simulink library "MarIn_blade"  (R2017a)
settings: Solver=VariableStepAuto  StartTime=0.0  StopTime=10.0  RelTol=1e-3
undefined symbols (not defined in the file or in its folder): bladePar, data_wind_mann, eta_init_n, g, k_t1, k_t2, k_w1, k_w2, lw2, m_h, meanWindSpeed, nu_init_b, p_h_dot_init, p_h_init, posCraneTip, posSling_b, posTuggerline_b, posTuggerlineBase_n, sigbuilder_block
undefined symbols (not defined in the file): d_w1, lt1_init
libraries: MarIn_blade x37
(part 1 of 2)
settings Model: Creator=zhengrur  LastModifiedBy=zhengrur

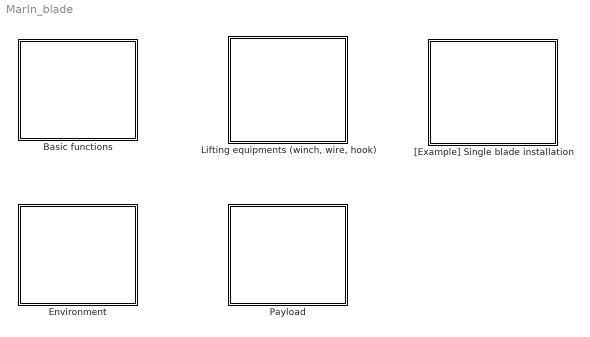
== system MarIn_blade ==
  Basic functions : Subsystem
  Environment : Subsystem
  "Lifting equipments (winch, wire, hook)" : Subsystem
  Payload : Subsystem
  "[Example] Single blade installation" : Subsystem  mask([Example] Single blade installation){}
      mask help:
      | This is an example to use the MarIn toolbox to model single blade installation.
      |
      | Author: Zhengru Ren
      | Date:  19/09/2017

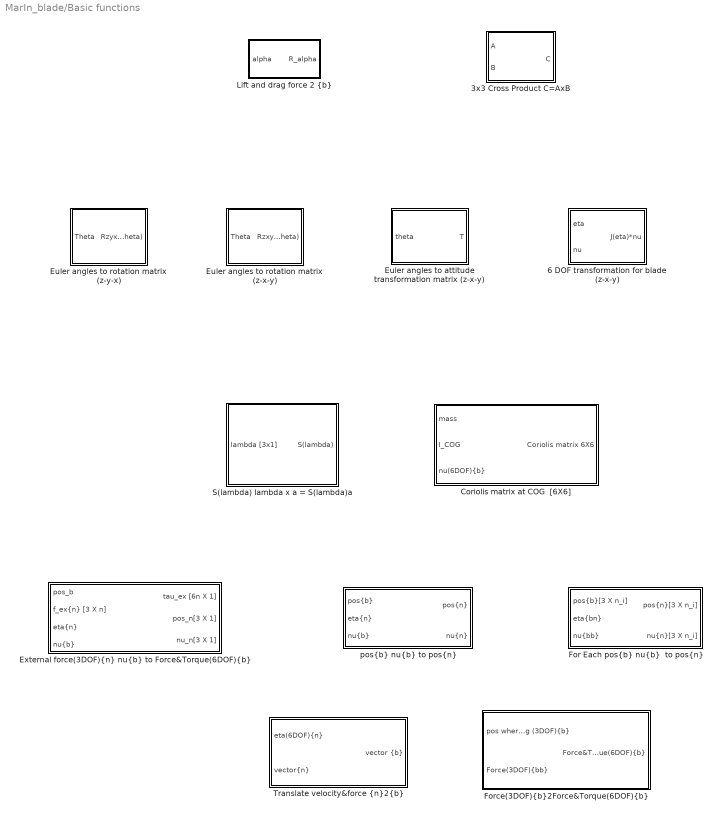
== system MarIn_blade/Basic functions ==
  3x3 Cross Product C=AxB : Subsystem  mask(3x3 Cross Product C=AxB){}
      mask help:
      | [3X1] vector cross product.
      |
      | Author: Zhengru Ren
      | Date: April 22, 2017
  6 DOF transformation for blade (z-x-y) : Subsystem  mask(6 DOF transformation for blade (z-x-y)){}
      mask help:
      | This is an example to use trasform body-fixed velocity to the global frame, with a z-x-y sequence.
      |
      | Author: Zhengru Ren
      | Date:  19/09/2017
  Coriolis matrix at COG  [6X6] : Subsystem  mask(Mass matrix at COG[6X6]){}
      mask help:
      | This block is used to generate the 6X6 mass matrix at the COG.
      |
      |
      | Author: Zhengru Ren
      | Date: April 20, 2017
  Euler angles to rotation matrix (z-x-y) : Subsystem  mask(Euler2R){}
      mask help: Determine the 3-by-3 rotation matrix from the Euler angles (pitch, roll, yaw) using the zxy convention.
      mask Display:
      | port_label('input',1,'theta')
      | port_label('output',1,'R_zxy')
  Euler angles to rotation matrix (z-y-x) : Subsystem  mask(Euler2R){}
      mask help: Determine the 3-by-3 rotation matrix from the Euler angles (roll, pitch, yaw) using the zyx convention.
      mask Display:
      | port_label('input',1,'Theta')
      | port_label('output',1,'R_zyx')
  Euler angles to attitude transformation matrix (z-x-y) : Subsystem  mask(Euler2T){}
      mask help: Determine the 3-by-3 attitude transformation matrix from the Euler angles (roll, pitch, yaw).
      mask Display:
      | port_label('input',1,'Theta')
      | port_label('output',1,'T_zxy')
  "External force(3DOF){n} nu{b} to Force&Torque(6DOF){b}" : Subsystem  mask(External force(3DOF){n} nu{b} to Force&Torque(6DOF){b}){}
      mask help:
      | Translate position and velocity in {b} to {n}.
      |
      |
      | Author: Zhengru Ren
      | Date: April 22, 2017
  "For Each pos{b} nu{b}  to pos{n}" : Subsystem  mask(For Each pos{b} nu{b}  to pos{n}){posCOG_b=bladePar.posCOG, n_i=bladePar.n_i}
      mask prompts: posCOG_b "Position COG {b}"; n_i "number of segment (n_i)"
      mask help:
      | Translate EACH position and velocity in {b} to {n}.
      |
      |
      | Author: Zhengru Ren
      | Date: April 22, 2017
  "Force(3DOF){b}2Force&Torque(6DOF){b}" : Subsystem  mask(Force(3DOF){bb}2Force&Torque(6DOF){bb}){posCOG_bb=bladePar.posCOG}
      mask prompts: posCOG_bb "Position COG {bb}"
      mask help:
      | This block is used to argument a 3DOF force vector to a 6DOF [force;torque] vector.
      |
      |
      |
      |
      | Author: Zhengru Ren
      | Date: April 20, 2017
  "Lift and drag force 2 {b}" : Subsystem  mask(Lift&drag{b}){}
      mask help:
      | The rotational matrix which transformed from the aerodyanmics coordinate to the body-fixed frame.
      |
      | Author: Zhengru Ren
      | Date: April 22, 2017
      mask Display:
      | port_label('input',1,'alpha')
      | port_label('output',1,'R_alpha')
  S(lambda) lambda x a = S(lambda)a : Subsystem  mask(Smatrix){}
      mask help:
      | Output a 3X3 S martix, such that lambda x a = S(lambda)a
      |
      | Author: Zhengru Ren
      | Date: May 10, 2016
  "Translate velocity&force {n}2{b}" : Subsystem  mask(Translate velocity&force {n}2{bb}){}
      mask help:
      | This block is used to transform a 3DOF velcotiy or force vector from {n} to {bb}.
      |
      |
      |
      |
      | Author: Zhengru Ren
      | Date: April 20, 2017
  "pos{b} nu{b} to pos{n}" : Subsystem  TreatAsAtomicUnit=on  mask(pos{bb} to pos{bn} and pos{n}){posCOG_bb=bladePar.posCOG}
      mask prompts: posCOG_bb "Position COG {bb}"
      mask help:
      | Translate the position in {bb} to {bn} and {n}
      |
      |
      | Author: Zhengru Ren
      | Date: April 22, 2017

== system MarIn_blade/Environment ==
  3D wind generator with Mann turbulence : Subsystem  mask(3D wind generator with Mann turbulence){turbulence_switch=on, posC_tb=[0,0,-90], angC_tb=[0,pi,pi/2], data_wind_mann=data_wind_mann}
      mask prompts: turbulence_switch "Turn on the turbulence"; posC_tb "Position of turbulence box center {n}  [X,Y,Z]"; angC_tb "Oritentations of the turbulence box {n} (rad)[phi,theta,psi]"; data_wind_mann "Mann model structure (run init_wind_mann)"
      mask help:
      | This module is used to simulate a wind with Mann turbulence generated from HAWC2 files.
      |
      | Remark: The tubulence will be significantly large if the initial position is not in the turbulence box. For more details, see revelant papers.
      |
      | Author: Zhengru Ren
      | Date: April 18, 2017
      mask Display:
      | image(imread('fig/turbulence.jpg'))
      | 
      | port_label('input', 1, 'Mean wind speed')
      | port_label('input', 2, 'Meansurement point{n}[N x 3]')
      | % port_label('input', 3, 'tau_wind{bb}')
      | 
      | port_label('output', 1, 'wind vel.(3DOF){n}')
      | % port_label('output', 2, 'nuCOG(6DOF){bb}')
      | % port_label('output', 3, 'pCOG(3DOF){n}')
      | % port_label('output', 4, 'pCOG_dot(3DOF){n}')
      | % port_label('output', 5, 'p_i(3DOF){n}')

== system MarIn_blade/Lifting equipments (winch, wire, hook) ==
  Hook : Subsystem  mask(Hook){m_h=m_h, p_h_init=p_h_init, p_h_dot_init=p_h_dot_init}
      mask prompts: m_h "Hook mass (m_h) [kg]"; p_h_init "Initial position of the hook"; p_h_dot_init "Initial velocity of the hook"
      mask help:
      | Used to simulate a hook.
      |
      | Author: Zhengru Ren
      | Date: May 20, 2016
      mask init:
      | invM_h = diag([1/m_h,1/m_h,1/m_h]);
  Winch : Subsystem  mask{l_0=lt1_init}
      mask prompts: l_0 "Initial rope length (m)"
  wire (changable length) : Subsystem  mask(Wire){k=k_w1, c=d_w1}
      mask prompts: k "stiffness (N/m)"; c "damping (Ns/m)"
      mask help:
      | Used to simulate a wire. Tension exists only when the enlongation is larger than 0.
      |
      |
      | Author: Zhengru Ren
      | Date: May 20, 2016
      mask DialogControl DescTextVar Prompt: %<MaskDescription>This module is applied to simulate an elastic rope. When the elongation < 0, there will be no restoring force.

== system MarIn_blade/Payload ==
  Suspended blade : Subsystem  mask(Blade){m_yoke=20e3, bladePar=bladePar, eta_init_n=eta_init_n, eta_init_b=nu_init_b, n_tugline=2, posTuggerline_b=posTuggerline_b, n_sling=2, posSling_b=posSling_b}
      mask prompts: m_yoke "Mass of yoke (kg)"; bladePar "Blade parameter structure"; eta_init_n "Initial position and attitude {n}"; eta_init_b "Initial velocity {b}"; n_tugline "Number of tugger lines (n_tugline)"; posTuggerline_b "Position of connection points to the Tuggerlines{b} [n_tugline x 3]"; n_sling "Number of slings (n_sling)"; posSling_b "Position of connection points to the slings {b} [3Xn_sling]"
      mask help:
      | This block is used to simulate a suspended blade lifted by a crane and control by tuglines.
      |
      |
      | Author: Zhengru Ren
      | Date: April 20, 2017
      mask init:
      | invM_total = inv(bladePar.M+diag([m_yoke,m_yoke,m_yoke,0,0,0]));
      mask Display:
      | image(imread('fig/blade.png'))
      | 
      | port_label('input', 1, 'f_sling1{n}')
      | port_label('input', 2, 'f_sling2{n}')
      | port_label('input', 3, 'f_tagline1{n}')
      | port_label('input', 4, 'f_tagline2{n}')
      | port_label('input', 5, 'tau_wind{b}')
      | 
      | port_label('output', 1, 'etaCOG(6DOF){n}')
      | port_label('output', 2, 'nuCOG(6DOF){b}')
      | port_label('output', 3, 'BUS')
  Wind loads acting on the blade : Subsystem  mask(Wind loads acting on the blade){}
      mask help:
      | This module is used to calculate the wind load acting on a blade in the body frame.
      |
      | Author: Zhengru Ren
      | Date: April 18, 2017
      mask Display:
      | image(imread('fig/blade_coordinate2.png'))
      | 
      | port_label('input', 1, 'eta_n')
      | port_label('input', 2, 'wind vel.{n}[3 x n_i]')
      | port_label('input', 3, 'nu_i{n}[3 x n_i]')
      | % port_label('input', 3, 'tau_wind{bb}')
      | 
      | port_label('output', 1, 'tau_wind{b}')
      | port_label('output', 2, 'BUS')
      | % port_label('output', 2, 'nuCOG(6DOF){bb}')
      | % port_label('output', 3, 'pCOG(3DOF){n}')
      | % port_label('output', 4, 'pCOG_dot(3DOF){n}')
      | % port_label('output', 5, 'p_i(3DOF){n}')

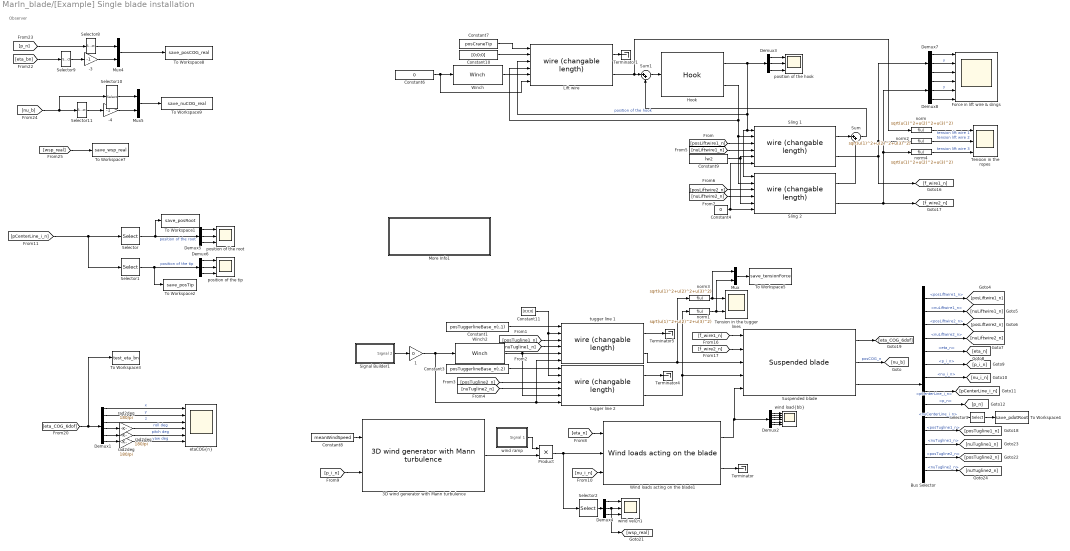
== system MarIn_blade/[Example] Single blade installation ==
  note: Observer
  " rad2deg" : Gain  Gain=180/pi
  -3 : Gain  Gain=-1
  -4 : Gain  Gain=-1
  1 : Gain  Gain=0
  3D wind generator with Mann turbulence : MarIn_blade/Environment/3D wind generator with Mann turbulence  turbulence_switch=on  posC_tb=[0,0,-90]  angC_tb=[0,0,0]  data_wind_mann=data_wind_mann
  Bus Selector : BusSelector  OutputSignals=posLiftwire1_n,nuLiftwire1_n,posLiftwire2_n,nuLiftwire2_n,eta_n,p_i_n,nu_i_n,pCenterLine_i_n,p_n,nuCenterLine_i_n,posTugline1_n,nuTugline1_n,posTugline2_n,nuTugline2_n
  Constant1 : Constant  Value=posTuggerlineBase_n(:,1)
  Constant10 : Constant  Value=[0;0;0]
  Constant11 : Constant  Value=[0;0;0]
  Constant3 : Constant  Value=posTuggerlineBase_n(:,2)
  Constant4 : Constant  Value=0
  Constant6 : Constant  Value=0
  Constant7 : Constant  Value=posCraneTip
  Constant8 : Constant  Value=meanWindSpeed
  Constant9 : Constant  Value=lw2
  Demux1 : Demux  Outputs=6
  Demux2 : Demux  Outputs=6
  Demux{3..8} (6 alike) : Demux  Outputs=3
  Force in lift wire & slings : Scope  NumInputPorts=6
  Hook : MarIn_blade/Lifting equipments (winch, wire, hook)/Hook  m_h=m_h  p_h_init=p_h_init  p_h_dot_init=p_h_dot_init
  Lift wire : MarIn_blade/Lifting equipments (winch, wire, hook)/wire (changable length)  k=k_w1  c=d_w1
  More Info1 : Subsystem
      settings: OpenFcn=run init_example_single_blade_installation.m
      mask Display: disp('Double-click to initialize the model')
  Mux : Mux  Inputs=2
  Mux4 : Mux  Inputs=2
  Mux5 : Mux  Inputs=2
  Product : Product
  Selector : Selector  NumberOfDimensions=2  InputPortWidth=3  IndexOptions=Index vector (dialog),Index vector (dialog)  Indices=[1 2 3],1  OutputSizes=1,1
  Selector1 : Selector  NumberOfDimensions=2  InputPortWidth=3  IndexOptions=Index vector (dialog),Index vector (dialog)  Indices=[1 2 3],bladePar.n_i  OutputSizes=1,1
  Selector10 : Selector  InputPortWidth=6  IndexOptions=Index vector (dialog)  Indices=[3,2]  OutputSizes=1
  Selector11 : Selector  InputPortWidth=6  IndexOptions=Index vector (dialog)  Indices=4  OutputSizes=1
  Selector2 : Selector  NumberOfDimensions=2  InputPortWidth=3  IndexOptions=Index vector (dialog),Index vector (dialog)  Indices=[1 2 3],20  OutputSizes=1,1
  Selector3 : Selector  NumberOfDimensions=2  InputPortWidth=3  IndexOptions=Index vector (dialog),Index vector (dialog)  Indices=[1 2 3],1  OutputSizes=1,1
  Selector8 : Selector  InputPortWidth=3  IndexOptions=Index vector (dialog)  Indices=[1 2]  OutputSizes=1
  Selector9 : Selector  InputPortWidth=6  IndexOptions=Index vector (dialog)  Indices=4  OutputSizes=1
  Signal Builder1 : Subsystem  Tag=STV Subsys  LoadFcn=sigbuilder_block('load');  StartFcn=sigbuilder_block('start');  StopFcn=sigbuilder_block('stop');  ClipboardFcn=sigbuilder_block('clipboard');  mask(Sigbuilder block){tuvar=[0:10]}
      mask help: Simulink:masks:SigbuilderBlock_MD
      mask init:
      | if ~strcmp(get_param(bdroot(gcbh),'SimulationStatus'),'stopped') tuvar = sigbuilder_block('maskInit'); end
      settings: CopyFcn=sigbuilder_block('copy');  DeleteFcn=sigbuilder_block('delete');  ModelCloseFcn=sigbuilder_block('modelClose');  PreSaveFcn=sigbuilder_block('preSave');  PauseFcn=sigbuilder_block('pause');  ContinueFcn=sigbuilder_block('continue');  NameChangeFcn=sigbuilder_block('namechange');  OpenFcn=sigbuilder_block('open',[6 30 1908 951.75 ]);  CloseFcn=sigbuilder_block('close');
      mask Display: plot(0, 0, 100, 100,[2, 2, 32, 32, 2], [68, 8, 8, 68, 68],[32, 2], [38, 38], [32, 19, 2],[53, 60, 44], [32, 17, 17, 2],[16, 16, 31, 31]);txt = getActiveGroup(gcbh);text(2, 100, txt,'verticalAlignment', 'top');
  Sling 1 : MarIn_blade/Lifting equipments (winch, wire, hook)/wire (changable length)  k=k_w2  c=d_w2
  Sling 2 : MarIn_blade/Lifting equipments (winch, wire, hook)/wire (changable length)  k=k_w2  c=d_w2
  Sum : Sum  Inputs=|++
  Sum1 : Sum  Inputs=|++
  Suspended blade : MarIn_blade/Payload/Suspended blade  m_yoke=20e3  bladePar=bladePar  eta_init_n=eta_init_n  eta_init_b=nu_init_b  n_tugline=2  posTuggerline_b=posTuggerline_b  n_sling=2  posSling_b=posSling_b
  Tension in the ropes : Scope  NumInputPorts=3
  Tension in the tugger lines : Scope  NumInputPorts=2
  Terminator{,1,4..5} (4 alike) : Terminator
  To Workspace1 : ToWorkspace  VariableName=save_posRoot  SaveFormat=Structure With Time  SampleTime=-1
  To Workspace2 : ToWorkspace  VariableName=save_posTip  SaveFormat=Structure With Time  SampleTime=-1
  To Workspace3 : ToWorkspace  VariableName=test_eta_bn  SaveFormat=Structure With Time  SampleTime=-1
  To Workspace4 : ToWorkspace  VariableName=save_pdotRoot  SaveFormat=Structure With Time  SampleTime=-1
  To Workspace5 : ToWorkspace  VariableName=save_tensionForce  SaveFormat=Structure With Time  SampleTime=-1
  To Workspace7 : ToWorkspace  VariableName=save_wsp_real  SaveFormat=Structure With Time  SampleTime=-1
  To Workspace8 : ToWorkspace  VariableName=save_posCOG_real  SaveFormat=Structure With Time  SampleTime=-1
  To Workspace9 : ToWorkspace  VariableName=save_nuCOG_real  SaveFormat=Structure With Time  SampleTime=-1
  Winch : MarIn_blade/Lifting equipments (winch, wire, hook)/Winch  l_0=lw1_init
  Winch2 : MarIn_blade/Lifting equipments (winch, wire, hook)/Winch  l_0=lt1_init
  Wind loads acting on the blade1 : MarIn_blade/Payload/Wind loads acting on the blade
      link override "Wind loads acting on node i/Lift and drag force 2 {b}": SourceBlock=MarIn_blade/Basic functions/Lift and drag force 2 {b}
  "etaCOG{n}" : Scope  NumInputPorts=6
  norm{,1..4} (5 alike) : Fcn  Expr=sqrt(u(1)^2+u(2)^2+u(3)^2)
  position of the hook : Scope  NumInputPorts=3
  position of the root : Scope  NumInputPorts=3
  position of the tip : Scope  NumInputPorts=3
  rad2deg : Gain  Gain=180/pi
  "rad2deg " : Gain  Gain=180/pi
  tugger line 1 : MarIn_blade/Lifting equipments (winch, wire, hook)/wire (changable length)  k=k_t1  c=d_t1
  tugger line 2 : MarIn_blade/Lifting equipments (winch, wire, hook)/wire (changable length)  k=k_t2  c=d_t2
  "wind load{bb}" : Scope  NumInputPorts=6
  wind ramp : Subsystem  Tag=STV Subsys  LoadFcn=sigbuilder_block('load');  StartFcn=sigbuilder_block('start');  StopFcn=sigbuilder_block('stop');  ClipboardFcn=sigbuilder_block('clipboard');  mask(Sigbuilder block){tuvar=[0:10]}
      mask help: Simulink:masks:SigbuilderBlock_MD
      mask init:
      | if ~strcmp(get_param(bdroot(gcbh),'SimulationStatus'),'stopped') tuvar = sigbuilder_block('maskInit'); end
      settings: CopyFcn=sigbuilder_block('copy');  DeleteFcn=sigbuilder_block('delete');  ModelCloseFcn=sigbuilder_block('modelClose');  PreSaveFcn=sigbuilder_block('preSave');  PauseFcn=sigbuilder_block('pause');  ContinueFcn=sigbuilder_block('continue');  NameChangeFcn=sigbuilder_block('namechange');  OpenFcn=sigbuilder_block('open',[6 30 1908 951.75 ]);  CloseFcn=sigbuilder_block('close');
      mask Display: plot(0, 0, 100, 100,[2, 2, 32, 32, 2], [68, 8, 8, 68, 68],[32, 2], [38, 38], [32, 19, 2],[53, 60, 44], [32, 17, 17, 2],[16, 16, 31, 31]);txt = getActiveGroup(gcbh);text(2, 100, txt,'verticalAlignment', 'top');
  "wind vel{n}" : Scope  NumInputPorts=3
  wires:
  Constant8/1 -> 3D wind generator with Mann turbulence/1
  Hook/2 -> Lift wire/4, Sling 2/2, Sling 1/2
  Sling 1/1 -> Sum/1
  Winch/1 -> Lift wire/5
  [eta_COG_6dof] -> To Workspace3/1, Demux1/1
  Demux1/5 -> rad2deg/1
  Demux1/4 -> "rad2deg "/1
  Demux2/1 -> "wind load{bb}"/1
  Demux2/2 -> "wind load{bb}"/2
  Demux2/3 -> "wind load{bb}"/3
  Wind loads acting on the blade1/2 -> Terminator/1
  Suspended blade/3 -> Bus Selector/1
  [p_i_n] -> 3D wind generator with Mann turbulence/2
  [posLiftwire1_n] -> Sling 1/3
  [eta_n] -> Wind loads acting on the blade1/1
  Sling 1/2 -> [f_wire1_n], Demux7/1, norm2/1
  [nuLiftwire1_n] -> Sling 1/4
  Suspended blade/2 -> [nu_b]  "posCOG_n"
  Demux2/4 -> "wind load{bb}"/4
  Demux2/5 -> "wind load{bb}"/5
  norm/1 -> Tension in the ropes/1  "tension lift wire 1"
  Demux2/6 -> "wind load{bb}"/6
  [nu_i_n] -> Wind loads acting on the blade1/3
  Sling 2/1 -> Sum/2
  Sling 2/2 -> [f_wire2_n], Demux8/1, norm4/1
  [posLiftwire2_n] -> Sling 2/3
  [nuLiftwire2_n] -> Sling 2/4
  Constant9/1 -> Sling 1/5, Sling 2/5
  Constant7/1 -> Lift wire/1
  Constant10/1 -> Lift wire/2
  Sum/1 -> Sum1/2
  Lift wire/2 -> norm/1, Sum1/1
  Lift wire/1 -> Terminator1/1
  Sum1/1 -> Hook/1
  norm2/1 -> Tension in the ropes/2  "tension lift wire 2"
  norm4/1 -> Tension in the ropes/3  "tension lift wire 3"
  Demux3/1 -> position of the hook/1
  Demux3/3 -> position of the hook/3
  Demux3/2 -> position of the hook/2
  Hook/1 -> Lift wire/3, Sling 2/1, Sling 1/1, Demux3/1  "position of the hook"
  Demux4/1 -> "wind vel{n}"/1
  Demux4/3 -> "wind vel{n}"/3
  Selector2/1 -> Demux4/1
  Demux5/1 -> position of the root/1
  Demux5/3 -> position of the root/3
  Demux5/2 -> position of the root/2
  Selector/1 -> Demux5/1, To Workspace1/1  "position of the root"
  Demux6/1 -> position of the tip/1
  Demux6/3 -> position of the tip/3
  Demux6/2 -> position of the tip/2
  Selector1/1 -> To Workspace2/1, Demux6/1  "position of the tip"
  Demux7/3 -> Force in lift wire & slings/3
  Demux7/2 -> Force in lift wire & slings/2  "y"
  Demux7/1 -> Force in lift wire & slings/1
  Demux8/3 -> Force in lift wire & slings/6
  Demux8/2 -> Force in lift wire & slings/5  "y"
  Demux8/1 -> Force in lift wire & slings/4
  [pCenterLine_i_n] -> Selector1/1, Selector/1
  Constant4/1 -> Sling 2/6, Sling 1/6
  Constant6/1 -> Lift wire/6, Winch/1
  Product/1 -> Wind loads acting on the blade1/2, Selector2/1
  wind ramp/1(Signal 1) -> Product/1
  Demux4/2 -> "wind vel{n}"/2, [wsp_real]
  tugger line 1/2 -> Suspended blade/3, norm3/1
  tugger line 2/2 -> Suspended blade/4, norm1/1
  Demux1/6 -> " rad2deg"/1
  Bus Selector/1 -> [posLiftwire1_n]  "<posLiftwire1_n>"
  Bus Selector/2 -> [nuLiftwire1_n]  "<nuLiftwire1_n>"
  Bus Selector/3 -> [posLiftwire2_n]  "<posLiftwire2_n>"
  Bus Selector/4 -> [nuLiftwire2_n]  "<nuLiftwire2_n>"
  Bus Selector/5 -> [eta_n]  "<eta_n>"
  Bus Selector/6 -> [p_i_n]  "<p_i_n>"
  Bus Selector/7 -> [nu_i_n]  "<nu_i_n>"
  Bus Selector/8 -> [pCenterLine_i_n]  "<pCenterLine_i_n>"
  Bus Selector/9 -> [p_n]  "<p_n>"
  [f_wire1_n] -> Suspended blade/1
  [f_wire2_n] -> Suspended blade/2
  Suspended blade/1 -> [eta_COG_6dof]
  Bus Selector/10 -> Selector3/1  "<nuCenterLine_i_n>"
  Selector3/1 -> To Workspace4/1
  Winch2/1 -> tugger line 2/5, tugger line 1/5
  Constant1/1 -> tugger line 1/1
  Constant3/1 -> tugger line 2/1
  Constant11/1 -> tugger line 2/2, tugger line 1/2
  Signal Builder1/1(Signal 2) -> 1/1
  1/1 -> Winch2/1, tugger line 2/6, tugger line 1/6
  Bus Selector/11 -> [posTugline1_n]  "<posTugline1_n>"
  Bus Selector/13 -> [posTugline2_n]  "<posTugline2_n>"
  Bus Selector/12 -> [nuTugline1_n]  "<nuTugline1_n>"
  Bus Selector/14 -> [nuTugline2_n]  "<nuTugline2_n>"
  [posTugline1_n] -> tugger line 1/3
  [nuTugline1_n] -> tugger line 1/4
  [posTugline2_n] -> tugger line 2/3
  [nuTugline2_n] -> tugger line 2/4
  tugger line 1/1 -> Terminator5/1
  tugger line 2/1 -> Terminator4/1
  norm3/1 -> Mux/1, Tension in the tugger lines/1
  norm1/1 -> Mux/2, Tension in the tugger lines/2
  Mux/1 -> To Workspace5/1
  Selector9/1 -> -3/1
  Selector8/1 -> Mux4/1
  -3/1 -> Mux4/2
  Selector10/1 -> Mux5/1
  Selector11/1 -> -4/1
  -4/1 -> Mux5/2
  Mux5/1 -> To Workspace9/1
  Mux4/1 -> To Workspace8/1
  [eta_bn] -> Selector9/1
  [p_n] -> Selector8/1
  [nu_b] -> Selector11/1, Selector10/1
  [wsp_real] -> To Workspace7/1
  3D wind generator with Mann turbulence/1 -> Product/2
  Demux1/2 -> "etaCOG{n}"/2  "y"
  Demux1/1 -> "etaCOG{n}"/1  "x"
  Demux1/3 -> "etaCOG{n}"/3  "z"
  "rad2deg "/1 -> "etaCOG{n}"/4  "roll deg"
  " rad2deg"/1 -> "etaCOG{n}"/6  "yaw deg"
  rad2deg/1 -> "etaCOG{n}"/5  "pitch deg"
  Wind loads acting on the blade1/1 -> Suspended blade/5, Demux2/1

== system MarIn_blade/Basic functions/3x3 Cross Product C=AxB ==
  A : Inport
  B : Inport  Port=2
  "A " : InportShadow
  "B " : InportShadow  Port=2
  Subsystem2 : Subsystem
  Subsystem3 : Subsystem
  Sum : Sum  Inputs=+|-  SaturateOnIntegerOverflow=on  InputSameDT=on  OutDataTypeStr=Inherit: Same as first input
  C : Outport
  wires:
  "B "/1 -> Subsystem3/2(B)
  "A "/1 -> Subsystem3/1(A)
  Sum/1 -> C/1
  B/1 -> Subsystem2/2(B)
  A/1 -> Subsystem2/1(A)
  Subsystem2/1(Out1) -> Sum/1
  Subsystem3/1(Out1) -> Sum/2

== system MarIn_blade/Basic functions/6 DOF transformation for blade (z-x-y) ==
  note: Theta
  note: v
  note: omega
  eta : Inport
  nu : Inport  Port=2
  Euler angles to rotation matrix (z-x-y) : MarIn_blade/Basic functions/Euler angles to rotation matrix (z-x-y)
      settings: SourceProductName=MarIn(Blade)
  Euler angles to attitude transformation matrix (z-x-y) : MarIn_blade/Basic functions/Euler angles to attitude transformation matrix (z-x-y)
      settings: SourceProductName=MarIn(Blade)
  Mux : Mux  Inputs=2
  Product : Product  Inputs=**  Multiplication=Matrix(*)  SaturateOnIntegerOverflow=on  OutDataTypeStr=Inherit: Same as first input
  Product1 : Product  Inputs=**  Multiplication=Matrix(*)  SaturateOnIntegerOverflow=on  OutDataTypeStr=Inherit: Same as first input
  Selector : Selector  InputPortWidth=6  IndexOptions=Index vector (dialog)  Indices=[4 5 6]  OutputSizes=1
  Selector1 : Selector  InputPortWidth=6  IndexOptions=Index vector (dialog)  Indices=[1 2 3]  OutputSizes=1
  Selector2 : Selector  InputPortWidth=6  IndexOptions=Index vector (dialog)  Indices=[4 5 6]  OutputSizes=1
  J(eta)*nu : Outport
  wires:
  Product/1 -> Mux/1
  Selector/1 -> Euler angles to attitude transformation matrix (z-x-y)/1, Euler angles to rotation matrix (z-x-y)/1
  eta/1 -> Selector/1
  Euler angles to rotation matrix (z-x-y)/1 -> Product/1
  nu/1 -> Selector1/1, Selector2/1
  Selector1/1 -> Product/2
  Selector2/1 -> Product1/2
  Euler angles to attitude transformation matrix (z-x-y)/1 -> Product1/1
  Mux/1 -> J(eta)*nu/1
  Product1/1 -> Mux/2

== system MarIn_blade/Basic functions/Coriolis matrix at COG  [6X6] ==
  mass : Inport
  I_COG : Inport  Port=2
  "nu(6DOF){b}" : Inport  Port=3
  Gain : Gain  Gain=-1
  Overwrite Values [1:3,1:3] : S-Function  FunctionName=sdspoverwrite  Parameters=ColSpan, ColStartMode, ColStartIndex, ColEndMode, ColEndIndex, RowSpan, RowStartMode, RowStartIndex, RowEndMode, RowEndIndex, OverWriteDiag, ConstValue, DiagSpan, DiagStartMode, DiagStartIndex, DiagEndMode, DiagEndIndex, valFrom2ndIP  SFunctionDeploymentMode=off  EnableBusSupport=off  mask(Overwrite Values){OverWriteDiag=Submatrix, valFrom2ndIP=Second input port, ConstValue=0, RowSpan=Range of rows, RowStartMode=Index, RowStartIndex=1, RowEndMode=Index, RowEndIndex=3, ColSpan=Range of columns, ColStartMode=Index, ColStartIndex=1, ColEndMode=Index, ColEndIndex=3, DiagSpan=Range of elements, DiagStartMode=Index, DiagStartIndex=1, DiagEndMode=Index, DiagEndIndex=3}
      mask prompts: OverWriteDiag "Overwrite:"; valFrom2ndIP "Source of overwriting value(s):"; ConstValue "Overwrite with:"; RowSpan "Row span:"; RowStartMode "Starting row:"; RowStartIndex "Starting row index:"; RowEndMode "Ending row:"; RowEndIndex "Ending row index:"; ColSpan "Column span:"; ColStartMode "Starting column:"; ColStartIndex "Starting column index:"; ColEndMode "Ending column:"; ColEndIndex "Ending column index:"; DiagSpan "Diagonal span:"; DiagStartMode "Starting element:"; DiagStartIndex "Starting element index:"; DiagEndMode "Ending element:"; DiagEndIndex "Ending element index:"
      mask help:
      | Overwrites a selected portion of the input matrix--either a submatrix, full diagonal, or a portion of the diagonal.
      | Specify overwriting values as follows:
      |   --Matrix with the same dimensions as the submatrix
      |   --Vector with the same length as the portion of the diagonal
      |   --Scalar constant with which to replace each element in the submatrix or diagonal portion.
      |
      | Treats unoriented (1-D) input vectors as column vectors.
      mask init:
      | [x1,y1,xc,yc,xmc,ymc,xi,yi] = dspblkoverwrite('icon');
      | if valFrom2ndIP == 1
      |   i1=1;
      |   s1='';
      | else
      |   i1=2;
      |   s1='V';
      | end;
      mask Help: eval('blocksethelp');
      mask TypeOptions OverWriteDiag: Submatrix | Diagonal
      mask Callback OverWriteDiag: dspblkoverwrite
      mask TypeOptions valFrom2ndIP: Specify via dialog | Second input port
      mask Callback valFrom2ndIP: dspblkoverwrite
      mask TypeOptions RowSpan: All rows | One row | Range of rows
      mask Callback RowSpan: dspblkoverwrite
      mask TypeOptions RowStartMode: First | Index | Offset from last | Last | Offset from middle | Middle
      mask Callback RowStartMode: dspblkoverwrite
      mask TypeOptions RowEndMode: Index | Offset from last | Last | Offset from middle | Middle
      mask Callback RowEndMode: dspblkoverwrite
      mask TypeOptions ColSpan: All columns | One column | Range of columns
      mask Callback ColSpan: dspblkoverwrite
      mask TypeOptions ColStartMode: First | Index | Offset from last | Last | Offset from middle | Middle
      mask Callback ColStartMode: dspblkoverwrite
      mask TypeOptions ColEndMode: Index | Offset from last | Last | Offset from middle | Middle
      mask Callback ColEndMode: dspblkoverwrite
      mask TypeOptions DiagSpan: All elements | One element | Range of elements
      mask Callback DiagSpan: dspblkoverwrite
      mask TypeOptions DiagStartMode: First | Index | Offset from last | Last | Offset from middle | Middle
      mask Callback DiagStartMode: dspblkoverwrite
      mask TypeOptions DiagEndMode: Index | Offset from last | Last | Offset from middle | Middle
      mask Callback DiagEndMode: dspblkoverwrite
      mask Display:
      | plot(x1,y1,xc,yc,xmc,ymc,xi,yi);
      | port_label('input',1,'A');
      | port_label('output',1,'B');
      | port_label('input',i1,s1);
  Overwrite Values [4:6,4:6] : S-Function  FunctionName=sdspoverwrite  Parameters=ColSpan, ColStartMode, ColStartIndex, ColEndMode, ColEndIndex, RowSpan, RowStartMode, RowStartIndex, RowEndMode, RowEndIndex, OverWriteDiag, ConstValue, DiagSpan, DiagStartMode, DiagStartIndex, DiagEndMode, DiagEndIndex, valFrom2ndIP  SFunctionDeploymentMode=off  EnableBusSupport=off  mask(Overwrite Values){OverWriteDiag=Submatrix, valFrom2ndIP=Second input port, ConstValue=0, RowSpan=Range of rows, RowStartMode=Index, RowStartIndex=4, RowEndMode=Index, RowEndIndex=6, ColSpan=Range of columns, ColStartMode=Index, ColStartIndex=4, ColEndMode=Index, ColEndIndex=6, DiagSpan=Range of elements, DiagStartMode=Index, DiagStartIndex=2, DiagEndMode=Index, DiagEndIndex=4}
      mask prompts: OverWriteDiag "Overwrite:"; valFrom2ndIP "Source of overwriting value(s):"; ConstValue "Overwrite with:"; RowSpan "Row span:"; RowStartMode "Starting row:"; RowStartIndex "Starting row index:"; RowEndMode "Ending row:"; RowEndIndex "Ending row index:"; ColSpan "Column span:"; ColStartMode "Starting column:"; ColStartIndex "Starting column index:"; ColEndMode "Ending column:"; ColEndIndex "Ending column index:"; DiagSpan "Diagonal span:"; DiagStartMode "Starting element:"; DiagStartIndex "Starting element index:"; DiagEndMode "Ending element:"; DiagEndIndex "Ending element index:"
      mask help:
      | Overwrites a selected portion of the input matrix--either a submatrix, full diagonal, or a portion of the diagonal.
      | Specify overwriting values as follows:
      |   --Matrix with the same dimensions as the submatrix
      |   --Vector with the same length as the portion of the diagonal
      |   --Scalar constant with which to replace each element in the submatrix or diagonal portion.
      |
      | Treats unoriented (1-D) input vectors as column vectors.
      mask init:
      | [x1,y1,xc,yc,xmc,ymc,xi,yi] = dspblkoverwrite('icon');
      | if valFrom2ndIP == 1
      |   i1=1;
      |   s1='';
      | else
      |   i1=2;
      |   s1='V';
      | end;
      mask Help: eval('blocksethelp');
      mask TypeOptions OverWriteDiag: Submatrix | Diagonal
      mask Callback OverWriteDiag: dspblkoverwrite
      mask TypeOptions valFrom2ndIP: Specify via dialog | Second input port
      mask Callback valFrom2ndIP: dspblkoverwrite
      mask TypeOptions RowSpan: All rows | One row | Range of rows
      mask Callback RowSpan: dspblkoverwrite
      mask TypeOptions RowStartMode: First | Index | Offset from last | Last | Offset from middle | Middle
      mask Callback RowStartMode: dspblkoverwrite
      mask TypeOptions RowEndMode: Index | Offset from last | Last | Offset from middle | Middle
      mask Callback RowEndMode: dspblkoverwrite
      mask TypeOptions ColSpan: All columns | One column | Range of columns
      mask Callback ColSpan: dspblkoverwrite
      mask TypeOptions ColStartMode: First | Index | Offset from last | Last | Offset from middle | Middle
      mask Callback ColStartMode: dspblkoverwrite
      mask TypeOptions ColEndMode: Index | Offset from last | Last | Offset from middle | Middle
      mask Callback ColEndMode: dspblkoverwrite
      mask TypeOptions DiagSpan: All elements | One element | Range of elements
      mask Callback DiagSpan: dspblkoverwrite
      mask TypeOptions DiagStartMode: First | Index | Offset from last | Last | Offset from middle | Middle
      mask Callback DiagStartMode: dspblkoverwrite
      mask TypeOptions DiagEndMode: Index | Offset from last | Last | Offset from middle | Middle
      mask Callback DiagEndMode: dspblkoverwrite
      mask Display:
      | plot(x1,y1,xc,yc,xmc,ymc,xi,yi);
      | port_label('input',1,'A');
      | port_label('output',1,'B');
      | port_label('input',i1,s1);
  Product1 : Product  Multiplication=Matrix(*)
  Product2 : Product
  S(lambda) lambda x a = S(lambda)a1 : MarIn_blade/Basic functions/S(lambda) lambda x a = S(lambda)a
      settings: SourceProductName=MarIn(Blade)
  S(lambda) lambda x a = S(lambda)a2 : MarIn_blade/Basic functions/S(lambda) lambda x a = S(lambda)a
      settings: SourceProductName=MarIn(Blade)
  Selector : Selector  InputPortWidth=6  IndexOptions=Index vector (dialog)  Indices=[1 2 3]  OutputSizes=1
  zeros : Constant  Value=zeros(6,6)
  Coriolis matrix 6X6 : Outport
  wires:
  Product1/1 -> S(lambda) lambda x a = S(lambda)a1/1
  Product2/1 -> Overwrite Values [1:3,1:3]/2
  S(lambda) lambda x a = S(lambda)a2/1 -> Product2/2
  mass/1 -> Product2/1
  I_COG/1 -> Product1/1
  "nu(6DOF){b}"/1 -> Selector/1
  Overwrite Values [1:3,1:3]/1 -> Overwrite Values [4:6,4:6]/1
  zeros/1 -> Overwrite Values [1:3,1:3]/1
  S(lambda) lambda x a = S(lambda)a1/1 -> Gain/1
  Overwrite Values [4:6,4:6]/1 -> Coriolis matrix 6X6/1
  Gain/1 -> Overwrite Values [4:6,4:6]/2
  Selector/1 -> S(lambda) lambda x a = S(lambda)a2/1, Product1/2  "omega"

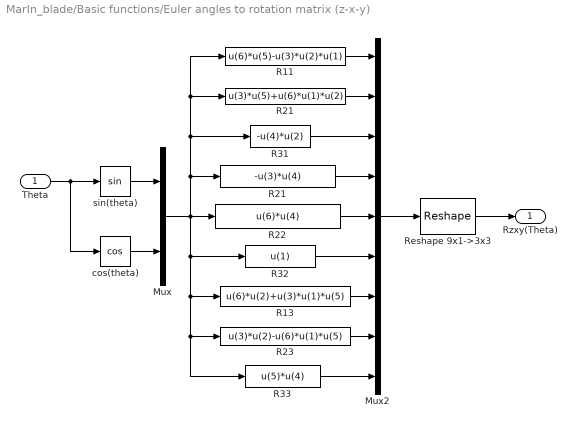
== system MarIn_blade/Basic functions/Euler angles to rotation matrix (z-x-y) ==
  Theta : Inport
  Mux : Mux  Inputs=2
  Mux2 : Mux  Inputs=9
  R11 : Fcn  Expr=u(6)*u(5)-u(3)*u(2)*u(1)
  R13 : Fcn  Expr=u(6)*u(2)+u(3)*u(1)*u(5)
  R21 : Fcn  Expr=-u(3)*u(4)
  "R21 " : Fcn  Expr=u(3)*u(5)+u(6)*u(1)*u(2)
  R22 : Fcn  Expr=u(6)*u(4)
  R23 : Fcn  Expr=u(3)*u(2)-u(6)*u(1)*u(5)
  "R31 " : Fcn  Expr=-u(4)*u(2)
  R32 : Fcn  Expr=u(1)
  R33 : Fcn  Expr=u(5)*u(4)
  Reshape 9x1->3x3 : Reshape  OutputDimensionality=Customize  OutputDimensions=[3,3]
  cos(theta) : Trigonometry  Operator=cos
  sin(theta) : Trigonometry
  Rzxy(Theta) : Outport  InitialOutput=0
  wires:
  R33/1 -> Mux2/9
  R32/1 -> Mux2/6
  "R21 "/1 -> Mux2/2
  "R31 "/1 -> Mux2/3
  R21/1 -> Mux2/4
  R22/1 -> Mux2/5
  R13/1 -> Mux2/7
  R23/1 -> Mux2/8
  Mux/1 -> R21/1, "R21 "/1, R11/1, "R31 "/1, R22/1, R23/1, R33/1, R13/1, R32/1
  Theta/1 -> cos(theta)/1, sin(theta)/1
  cos(theta)/1 -> Mux/2
  sin(theta)/1 -> Mux/1
  Reshape 9x1->3x3/1 -> Rzxy(Theta)/1
  Mux2/1 -> Reshape 9x1->3x3/1
  R11/1 -> Mux2/1

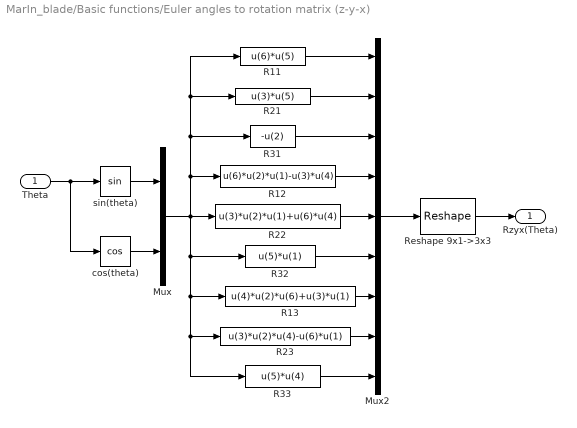
== system MarIn_blade/Basic functions/Euler angles to rotation matrix (z-y-x) ==
  Theta : Inport
  Mux : Mux  Inputs=2
  Mux2 : Mux  Inputs=9
  R11 : Fcn  Expr=u(6)*u(5)
  R12 : Fcn  Expr=u(6)*u(2)*u(1)-u(3)*u(4)
  R13 : Fcn  Expr=u(4)*u(2)*u(6)+u(3)*u(1)
  "R21 " : Fcn  Expr=u(3)*u(5)
  R22 : Fcn  Expr=u(3)*u(2)*u(1)+u(6)*u(4)
  R23 : Fcn  Expr=u(3)*u(2)*u(4)-u(6)*u(1)
  "R31 " : Fcn  Expr=-u(2)
  R32 : Fcn  Expr=u(5)*u(1)
  R33 : Fcn  Expr=u(5)*u(4)
  Reshape 9x1->3x3 : Reshape  OutputDimensionality=Customize  OutputDimensions=[3,3]
  cos(theta) : Trigonometry  Operator=cos
  sin(theta) : Trigonometry
  Rzyx(Theta) : Outport  InitialOutput=0
  wires:
  R33/1 -> Mux2/9
  R32/1 -> Mux2/6
  "R21 "/1 -> Mux2/2
  "R31 "/1 -> Mux2/3
  R12/1 -> Mux2/4
  R22/1 -> Mux2/5
  R13/1 -> Mux2/7
  R23/1 -> Mux2/8
  Mux/1 -> R12/1, "R21 "/1, R11/1, "R31 "/1, R22/1, R23/1, R33/1, R13/1, R32/1
  Theta/1 -> cos(theta)/1, sin(theta)/1
  cos(theta)/1 -> Mux/2
  sin(theta)/1 -> Mux/1
  Reshape 9x1->3x3/1 -> Rzyx(Theta)/1
  Mux2/1 -> Reshape 9x1->3x3/1
  R11/1 -> Mux2/1

== system MarIn_blade/Basic functions/Euler angles to attitude transformation matrix (z-x-y) ==
  theta : Inport
  Constant : Constant
  "Constant " : Constant  Value=0
  Mux2 : Mux  Inputs=9
  Reshape 9x1->3x3 : Reshape  OutputDimensionality=Customize  OutputDimensions=[3,3]
  T11 : Fcn  Expr=cos(u(2))
  T12 : Fcn  Expr=tan(u(1))*sin(u(2))
  T13 : Fcn  Expr=-sin(u(2))/cos(u(1))
  T31 : Fcn  Expr=sin(u(2))
  T32 : Fcn  Expr=-cos(u(2))*tan(u(1))
  T33 : Fcn  Expr=cos(u(2))/cos(u(1))
  T : Outport  InitialOutput=0
  wires:
  theta/1 -> T33/1, T32/1, T31/1, T13/1, T12/1, T11/1
  Reshape 9x1->3x3/1 -> T/1
  Mux2/1 -> Reshape 9x1->3x3/1
  T11/1 -> Mux2/1
  T12/1 -> Mux2/2
  T13/1 -> Mux2/3
  "Constant "/1 -> Mux2/6, Mux2/4
  Constant/1 -> Mux2/5
  T32/1 -> Mux2/8
  T33/1 -> Mux2/9
  T31/1 -> Mux2/7

== system MarIn_blade/Basic functions/External force(3DOF){n} nu{b} to Force&Torque(6DOF){b} ==
  pos_b : Inport
  "f_ex{n} [3 X n]" : Inport  Port=2
  "eta{n}" : Inport  Port=3
  "nu{b}" : Inport  Port=4
  "Force(3DOF){b}2Force&Torque(6DOF){b}" : MarIn_blade/Basic functions/Force(3DOF){b}2Force&Torque(6DOF){b}  posCOG_bb=bladePar.posCOG
      settings: SourceProductName=MarIn(Blade)
  "Translate velocity&force {n}2{b}" : MarIn_blade/Basic functions/Translate velocity&force {n}2{b}
      settings: SourceProductName=MarIn(Blade)
  "pos{b} nu{b} to pos{n}" : MarIn_blade/Basic functions/pos{b} nu{b} to pos{n}  posCOG_bb=bladePar.posCOG
      settings: SourceProductName=MarIn(Blade)
  tau_ex [6n X 1] : Outport
  pos_n[3 X 1] : Outport  Port=2
  nu_n[3 X 1] : Outport  Port=3
  wires:
  "eta{n}"/1 -> "Translate velocity&force {n}2{b}"/1, "pos{b} nu{b} to pos{n}"/2
  "f_ex{n} [3 X n]"/1 -> "Translate velocity&force {n}2{b}"/2
  "Force(3DOF){b}2Force&Torque(6DOF){b}"/1 -> tau_ex [6n X 1]/1
  "Translate velocity&force {n}2{b}"/1 -> "Force(3DOF){b}2Force&Torque(6DOF){b}"/2  "External force{bb}"
  pos_b/1 -> "Force(3DOF){b}2Force&Torque(6DOF){b}"/1, "pos{b} nu{b} to pos{n}"/1
  "pos{b} nu{b} to pos{n}"/1 -> pos_n[3 X 1]/1
  "nu{b}"/1 -> "pos{b} nu{b} to pos{n}"/3
  "pos{b} nu{b} to pos{n}"/2 -> nu_n[3 X 1]/1

== system MarIn_blade/Basic functions/For Each pos{b} nu{b}  to pos{n} ==
  "pos{b}[3 X n_i]" : Inport
  "eta{bn}" : Inport  Port=2
  "nu{bb}" : Inport  Port=3
  Reshape2 : Reshape  OutputDimensionality=Customize  OutputDimensions=[3,n_i]
  Reshape3 : Reshape  OutputDimensionality=Customize  OutputDimensions=[3,n_i]
  "pos{b} nu{b} to pos{n}" : Subsystem  TreatAsAtomicUnit=on  mask(pos{bb} to pos{bn} and pos{n}){posCOG_bb=bladePar.posCOG}
      mask prompts: posCOG_bb "Position COG {bb}"
      mask help:
      | Translate the position in {bb} to {bn} and {n}
      |
      |
      | Author: Zhengru Ren
      | Date: April 22, 2017
  "pos{n}[3 X n_i]" : Outport
  "nu{n}[3 X n_i]" : Outport  Port=2
  wires:
  "eta{bn}"/1 -> "pos{b} nu{b} to pos{n}"/2("eta{n}")
  "nu{bb}"/1 -> "pos{b} nu{b} to pos{n}"/3("nu{b}")
  "pos{b} nu{b} to pos{n}"/1("pos{n}") -> Reshape2/1  "[3n_i X 1]"
  "pos{b} nu{b} to pos{n}"/2("nu{n}") -> Reshape3/1  "[3n_i X 1]"
  "pos{b}[3 X n_i]"/1 -> "pos{b} nu{b} to pos{n}"/1("pos{b}")
  Reshape2/1 -> "pos{n}[3 X n_i]"/1
  Reshape3/1 -> "nu{n}[3 X n_i]"/1

== system MarIn_blade/Basic functions/Force(3DOF){b}2Force&Torque(6DOF){b} ==
  "pos where Force acting (3DOF){b}" : Inport
  "Force(3DOF){bb}" : Inport  Port=2
  3x3 Cross Product C=AxB : Subsystem
  Mux1 : Mux  Inputs=2
  Sum4 : Sum  Inputs=|+-
  "[0;0;0]1" : Constant  Value=posCOG_bb
  "Force&Torque(6DOF){b}" : Outport
  wires:
  Sum4/1 -> 3x3 Cross Product C=AxB/1(A)
  Mux1/1 -> "Force&Torque(6DOF){b}"/1
  "[0;0;0]1"/1 -> Sum4/2
  "pos where Force acting (3DOF){b}"/1 -> Sum4/1
  3x3 Cross Product C=AxB/1(C) -> Mux1/2
  "Force(3DOF){bb}"/1 -> 3x3 Cross Product C=AxB/2(B), Mux1/1

== system MarIn_blade/Basic functions/Lift and drag force 2 {b} ==
  alpha : Inport
  -1 : Gain  Gain=-1
  Mux1 : Mux
  Reshape 4x1->2x2 : Reshape  OutputDimensionality=Customize  OutputDimensions=[2,2]
  cos(theta) : Trigonometry  Operator=cos
  sin(theta) : Trigonometry
  R_alpha : Outport  InitialOutput=0
  wires:
  Reshape 4x1->2x2/1 -> R_alpha/1
  sin(theta)/1 -> Mux1/2, -1/1
  cos(theta)/1 -> Mux1/4, Mux1/1
  alpha/1 -> sin(theta)/1, cos(theta)/1
  Mux1/1 -> Reshape 4x1->2x2/1
  -1/1 -> Mux1/3

== system MarIn_blade/Basic functions/S(lambda) lambda x a = S(lambda)a ==
  lambda [3x1] : Inport
  Constant : Constant  Value=0
  Mux : Mux  Inputs=9
  Reshape 9x1->3x3 : Reshape  OutputDimensionality=Customize  OutputDimensions=[3,3]
  "S12 " : Fcn  Expr=-u(3)
  S13 : Fcn  Expr=u(2)
  S21 : Fcn  Expr=u(3)
  S23 : Fcn  Expr=-u(1)
  S31 : Fcn  Expr=-u(2)
  S32 : Fcn  Expr=u(1)
  S(lambda) : Outport
  wires:
  S23/1 -> Mux/8
  S13/1 -> Mux/7
  S32/1 -> Mux/6
  "S12 "/1 -> Mux/4
  Mux/1 -> Reshape 9x1->3x3/1
  Reshape 9x1->3x3/1 -> S(lambda)/1
  S21/1 -> Mux/2
  Constant/1 -> Mux/1, Mux/5, Mux/9
  lambda [3x1]/1 -> "S12 "/1, S31/1, S21/1, S32/1, S23/1, S13/1
  S31/1 -> Mux/3

== system MarIn_blade/Basic functions/Translate velocity&force {n}2{b} ==
  "eta(6DOF){n}" : Inport
  "vector{n}" : Inport  Port=2
  Euler angles to rotation matrix (z-x-y) : MarIn_blade/Basic functions/Euler angles to rotation matrix (z-x-y)
      settings: SourceProductName=MarIn(Blade)
  Math Function1 : Math  Operator=transpose  SaturateOnIntegerOverflow=on
  Product2 : Product  Multiplication=Matrix(*)
  Selector : Selector  InputPortWidth=6  IndexOptions=Index vector (dialog)  Indices=[4 5 6]  OutputSizes=1
  "vector {b}" : Outport
  wires:
  Selector/1 -> Euler angles to rotation matrix (z-x-y)/1  "Theta"
  Math Function1/1 -> Product2/1  "{n}2{b}"
  Euler angles to rotation matrix (z-x-y)/1 -> Math Function1/1
  "eta(6DOF){n}"/1 -> Selector/1
  Product2/1 -> "vector {b}"/1
  "vector{n}"/1 -> Product2/2

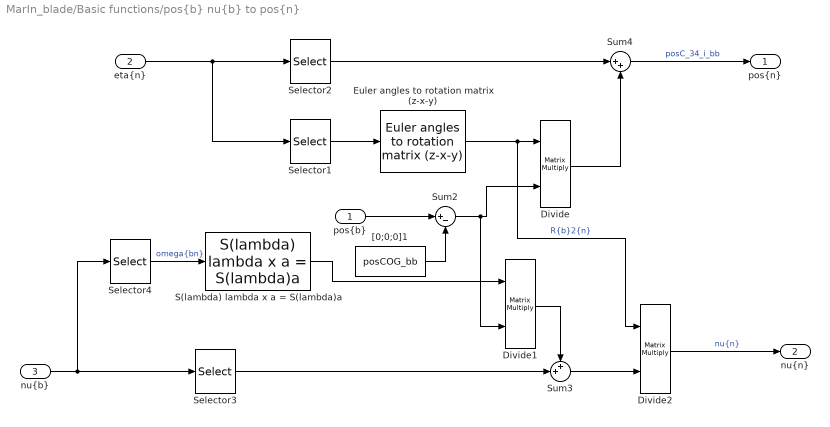
== system MarIn_blade/Basic functions/pos{b} nu{b} to pos{n} ==
  "pos{b}" : Inport
  "eta{n}" : Inport  Port=2
  "nu{b}" : Inport  Port=3
  Divide : Product  Inputs=**  Multiplication=Matrix(*)
  Divide1 : Product  Multiplication=Matrix(*)
  Divide2 : Product  Multiplication=Matrix(*)
  Euler angles to rotation matrix (z-x-y) : MarIn_blade/Basic functions/Euler angles to rotation matrix (z-x-y)
      settings: SourceProductName=MarIn(Blade)
  S(lambda) lambda x a = S(lambda)a : MarIn_blade/Basic functions/S(lambda) lambda x a = S(lambda)a
      settings: SourceProductName=MarIn (Blade)
  Selector1 : Selector  InputPortWidth=6  IndexOptions=Index vector (dialog)  Indices=[4 5 6]  OutputSizes=1
  Selector2 : Selector  InputPortWidth=6  IndexOptions=Index vector (dialog)  Indices=[1 2 3]  OutputSizes=1
  Selector3 : Selector  InputPortWidth=6  IndexOptions=Index vector (dialog)  Indices=[1 2 3]  OutputSizes=1
  Selector4 : Selector  InputPortWidth=6  IndexOptions=Index vector (dialog)  Indices=[4 5 6]  OutputSizes=1
  Sum2 : Sum  Inputs=|+-
  Sum3 : Sum  Inputs=++|
  Sum4 : Sum  Inputs=|++
  "[0;0;0]1" : Constant  Value=posCOG_bb
  "pos{n}" : Outport
  "nu{n}" : Outport  Port=2
  wires:
  S(lambda) lambda x a = S(lambda)a/1 -> Divide1/1
  Divide1/1 -> Sum3/1
  Sum3/1 -> Divide2/2
  "[0;0;0]1"/1 -> Sum2/2
  Sum2/1 -> Divide/2, Divide1/2
  Divide2/1 -> "nu{n}"/1  "nu{n}"
  Selector3/1 -> Sum3/2
  "nu{b}"/1 -> Selector4/1, Selector3/1
  "pos{b}"/1 -> Sum2/1
  Divide/1 -> Sum4/2
  Euler angles to rotation matrix (z-x-y)/1 -> Divide2/1, Divide/1  "R{b}2{n}"
  Selector2/1 -> Sum4/1
  "eta{n}"/1 -> Selector2/1, Selector1/1
  Sum4/1 -> "pos{n}"/1  "posC_34_i_bb"
  Selector1/1 -> Euler angles to rotation matrix (z-x-y)/1
  Selector4/1 -> S(lambda) lambda x a = S(lambda)a/1  "omega{bn}"

== system MarIn_blade/Environment/3D wind generator with Mann turbulence ==
  Mean wind speed : Inport
  "measurement position {n} [NX3]" : Inport  Port=2
  Reshape1 : Reshape  OutputDimensionality=Customize  OutputDimensions=[3,length(bladePar.chordLength_i)]
  Subsystem : Subsystem
  "wind vel. {n}" : Outport
  wires:
  Mean wind speed/1 -> Subsystem/1(Mean wind speed)
  "measurement position {n} [NX3]"/1 -> Subsystem/2("measurement position {n} [NX3]")
  Subsystem/1("wind vel. {n}") -> Reshape1/1
  Reshape1/1 -> "wind vel. {n}"/1

== system MarIn_blade/Lifting equipments (winch, wire, hook)/Hook ==
  total external force : Inport
  Integrator2 : Integrator  InitialCondition=p_h_dot_init
  Integrator3 : Integrator  InitialCondition=p_h_init
  Sum6 : Sum
  hook gravity : Constant  Value=[0;0;m_h*g]
  invM_h : Gain  Gain=invM_h  Multiplication=Matrix(K*u)
  posHook : Outport
  velHook : Outport  Port=2
  wires:
  Integrator2/1 -> velHook/1, Integrator3/1  "p_h_dot"
  total external force/1 -> Sum6/1
  hook gravity/1 -> Sum6/2
  invM_h/1 -> Integrator2/1  "p_h_ddot"
  Sum6/1 -> invM_h/1
  Integrator3/1 -> posHook/1  "p_h"

== system MarIn_blade/Lifting equipments (winch, wire, hook)/Winch ==
  winch speed : Inport
  Integrator1 : Integrator  InitialCondition=l_0
  l_c1 : Outport
  wires:
  winch speed/1 -> Integrator1/1
  Integrator1/1 -> l_c1/1

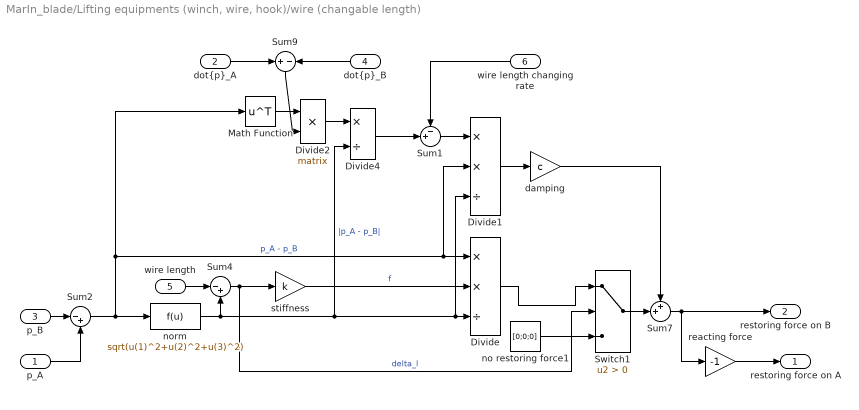
== system MarIn_blade/Lifting equipments (winch, wire, hook)/wire (changable length) ==
  p_A : Inport
  "dot{p}_A" : Inport  Port=2
  p_B : Inport  Port=3
  "dot{p}_B" : Inport  Port=4
  wire length : Inport  Port=5
  wire length changing rate : Inport  Port=6
  Divide : Product  Inputs=**/
  Divide1 : Product  Inputs=**/
  Divide2 : Product  Inputs=**  Multiplication=Matrix(*)
  Divide4 : Product  Inputs=*/
  Math Function : Math  Operator=transpose  SaturateOnIntegerOverflow=on
  Sum1 : Sum  Inputs=-+|
  Sum2 : Sum  Inputs=|-+
  Sum4 : Sum  Inputs=|-+
  Sum7 : Sum  Inputs=++|
  Sum9 : Sum  Inputs=+|-
  Switch1 : Switch  Criteria=u2 > Threshold
  damping : Gain  Gain=c
  no restoring force1 : Constant  Value=[0;0;0]
  norm : Fcn  Expr=sqrt(u(1)^2+u(2)^2+u(3)^2)
  reacting force : Gain  Gain=-1
  stiffness : Gain  Gain=k
  restoring force on A : Outport
  restoring force on B : Outport  Port=2
  wires:
  Sum9/1 -> Divide2/2
  wire length changing rate/1 -> Sum1/1
  Sum1/1 -> Divide1/1
  Divide4/1 -> Sum1/2
  Divide2/1 -> Divide4/1
  Math Function/1 -> Divide2/1
  damping/1 -> Sum7/1
  Divide1/1 -> damping/1
  stiffness/1 -> Divide/2  "f"
  no restoring force1/1 -> Switch1/3
  p_A/1 -> Sum2/2
  Sum4/1 -> Switch1/2, stiffness/1  "delta_l"
  "dot{p}_A"/1 -> Sum9/1
  "dot{p}_B"/1 -> Sum9/2
  Sum7/1 -> reacting force/1, restoring force on B/1
  wire length/1 -> Sum4/1
  Sum2/1 -> Math Function/1, Divide/1, Divide1/2, norm/1  "p_A - p_B"
  norm/1 -> Sum4/2, Divide/3, Divide1/3, Divide4/2  "|p_A - p_B|"
  p_B/1 -> Sum2/1
  reacting force/1 -> restoring force on A/1
  Divide/1 -> Switch1/1
  Switch1/1 -> Sum7/2
